simulink model "SimpleGeomMdlGreenHouseOptimization"  (R2015a)
settings: Solver=ode45  StartTime=StartTimeSimulation  StopTime=EndTimeSimulation  MaxStep=1  RelTol=1e-3
settings Model: SimulationMode=accelerator  CovSFcnEnable=off  Creator=Oleg_2  LastModifiedBy=Oleg
settings DataIOCC: ExternalInput=inputSignal  LimitDataPoints=off  LoadExternalInput=on  SaveCompleteFinalSimState=on  SaveFormat=StructureWithTime  SignalLogging=off  DSMLogging=off  VisualizeSimOutput=off  SaveTime=off
settings DebuggingCC: UnderspecifiedInitializationDetection=Classic  MergeDetectMultiDrivingBlocksExec=none  SolverPrmCheckMsg=warning  InheritedTsInSrcMsg=none  ModelReferenceExtraNoncontSigs=warning

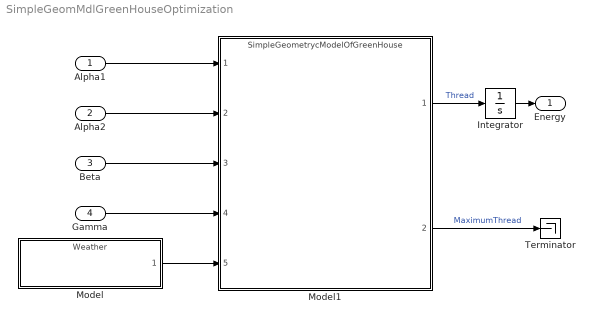
== system SimpleGeomMdlGreenHouseOptimization ==
  Alpha1 : Inport  OutDataTypeStr=double  PortDimensions=1  SampleTime=0
  Alpha2 : Inport  Port=2  OutDataTypeStr=double  PortDimensions=1  SampleTime=0
  Beta : Inport  Port=3  OutDataTypeStr=double  PortDimensions=1  SampleTime=0
  Gamma : Inport  Port=4  OutDataTypeStr=double  PortDimensions=1  SampleTime=0
  Integrator : Integrator
  Model : ModelReference  ModelNameDialog=Weather.slx  SimulationMode=Normal  ModelReferenceVersion=1.52  CopyOfModelName=Weather.slx  DefaultDataLogging=on
  Model1 : ModelReference  ModelNameDialog=SimpleGeometrycModelOfGreenHouse.slx  SimulationMode=Normal  ModelReferenceVersion=1.37  CopyOfModelName=SimpleGeometrycModelOfGreenHouse.slx  DefaultDataLogging=on
  Terminator : Terminator
  Energy : Outport
  wires:
  Model1/1 -> Integrator/1  "Thread"
  Integrator/1 -> Energy/1
  Model1/2 -> Terminator/1  "MaximumThread"
  Gamma/1 -> Model1/4
  Beta/1 -> Model1/3
  Alpha2/1 -> Model1/2
  Alpha1/1 -> Model1/1
  Model/1 -> Model1/5
